simulink model "rot_kin"  (R2019b)
settings: Solver=VariableStepAuto  StartTime=0.0  StopTime=40  RelTol=1e-3
libraries: sharedtransform x3, aerolibutil x1, sharedutil x1
settings Model: Creator=benma  LastModifiedBy=benma
settings DataIOCC: ReturnWorkspaceOutputs=off
settings DebuggingCC: ArithmeticOperatorsInVariantConditions=warning
settings SFSimCC: CustomCodeUndefinedFunction=UseInterfaceOnly

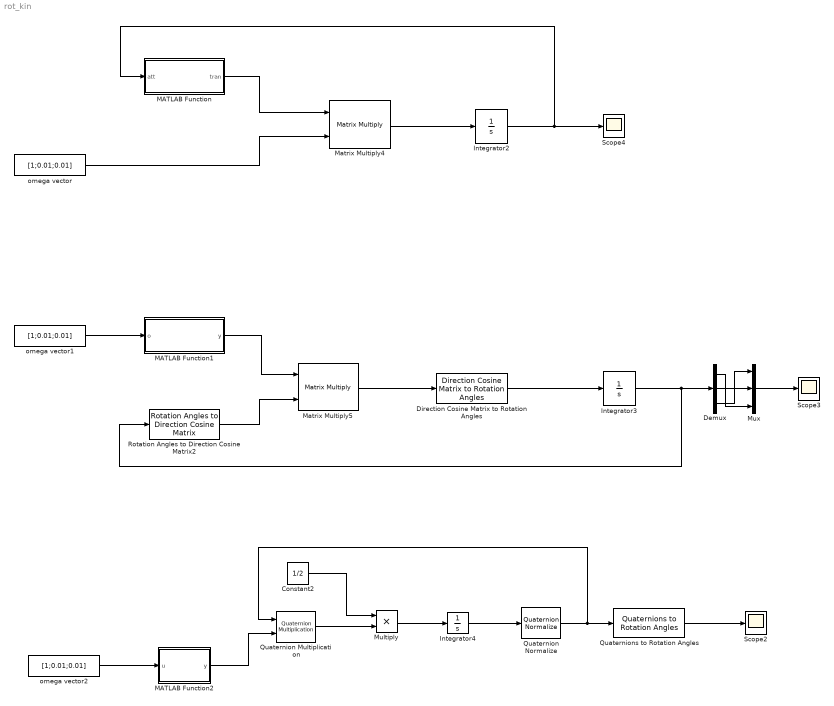
== system rot_kin ==
  Constant2 : Constant  Value=1/2
  Demux : Demux  Outputs=3
  Direction Cosine Matrix to Rotation Angles : sharedtransform/Direction Cosine Matrix to Rotation Angles  rotationOrder=ZYX  aMode=aMode  action=None  tolerance=eps(2)
      settings: SourceProductName=Aerospace Blockset  SourceProductBaseCode=AE
  Integrator2 : Integrator  InitialCondition=[0;0;0]
  Integrator3 : Integrator
  Integrator4 : Integrator  InitialCondition=[1;0;0;0]
  MATLAB Function : MATLAB Function  TreatAsAtomicUnit=on
  MATLAB Function1 : MATLAB Function  TreatAsAtomicUnit=on
  MATLAB Function2 : MATLAB Function  TreatAsAtomicUnit=on
  Matrix Multiply4 : Product  Multiplication=Matrix(*)
  Matrix Multiply5 : Product  Multiplication=Matrix(*)
  Multiply : Product
  Mux : Mux  Inputs=3
  Quaternion Multiplication : aerolibutil/Quaternion Multiplication
  Quaternion Normalize : sharedutil/Quaternion Normalize  aMode=aMode
      settings: SourceProductName=Aerospace Blockset  SourceProductBaseCode=AE
  Quaternions to Rotation Angles : sharedtransform/Quaternions to Rotation Angles  rotationOrder=ZYX  aMode=aMode
      settings: SourceProductBaseCode=AE
  Rotation Angles to Direction Cosine Matrix2 : sharedtransform/Rotation Angles to Direction Cosine Matrix  rotationOrder=ZYX  aMode=aMode
      settings: SourceProductBaseCode=AE
  Scope2 : Scope
  Scope3 : Scope
  Scope4 : Scope
  omega vector : Constant  Value=[1;0.01;0.01]
  omega vector1 : Constant  Value=[1;0.01;0.01]
  omega vector2 : Constant  Value=[1;0.01;0.01]
  wires:
  omega vector/1 -> Matrix Multiply4/2
  MATLAB Function/1(tran) -> Matrix Multiply4/1
  Matrix Multiply4/1 -> Integrator2/1
  Integrator2/1 -> Scope4/1, MATLAB Function/1(att)
  Integrator3/1 -> Demux/1, Rotation Angles to Direction Cosine Matrix2/1
  omega vector1/1 -> MATLAB Function1/1(o)
  MATLAB Function1/1(y) -> Matrix Multiply5/1
  Rotation Angles to Direction Cosine Matrix2/1 -> Matrix Multiply5/2
  Matrix Multiply5/1 -> Direction Cosine Matrix to Rotation Angles/1
  Direction Cosine Matrix to Rotation Angles/1 -> Integrator3/1
  Constant2/1 -> Multiply/1
  Quaternion Multiplication/1 -> Multiply/2
  Multiply/1 -> Integrator4/1
  Integrator4/1 -> Quaternion Normalize/1
  Quaternion Normalize/1 -> Quaternion Multiplication/1, Quaternions to Rotation Angles/1
  Quaternions to Rotation Angles/1 -> Scope2/1
  omega vector2/1 -> MATLAB Function2/1(u)
  MATLAB Function2/1(y) -> Quaternion Multiplication/2
  Demux/2 -> Mux/2
  Demux/3 -> Mux/1
  Demux/1 -> Mux/3
  Mux/1 -> Scope3/1

== matlab function rot_kin/MATLAB Function1 ==
  data: y output; o input
function y = fcn(o)
% o = (p;q;r)
omega = [0 -o(1) o(3);o(1) 0 -o(2);-o(3) o(2) 0];
y = omega;

== matlab function rot_kin/MATLAB Function ==
  data: tran output; att input
function tran = att2tran(att)
% att = [phi;theta;psi]
tran = [1 tan(att(2))*sin(att(1)) tan(att(2))*cos(att(1));0 cos(att(1)) -sin(att(1));0 sin(att(1))/cos(att(2)) cos(att(1))/cos(att(2))];
edn

== matlab function rot_kin/MATLAB Function2 ==
  data: u input; y output
function y = makeq(u)
v = [0;u(1);u(2);u(3)];
y = v;
